simulink model "carac_RPM"  (R2022b)
settings: Solver=VariableStepAuto  StartTime=0.0  StopTime=inf  RelTol=1e-3
libraries: robotlib x3
settings Model: Creator=guillermo  LastModifiedBy=alex

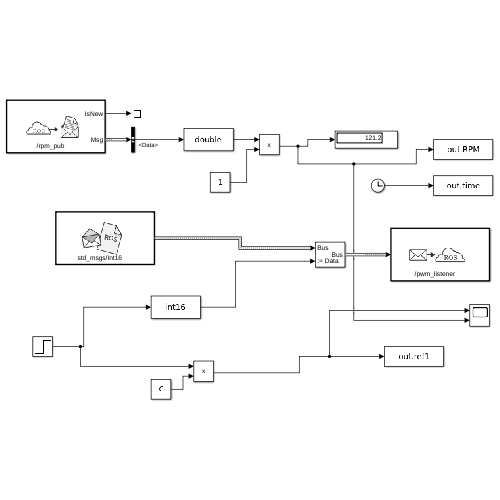
[thumbnail: Simulink's stored preview of the top-level diagram]
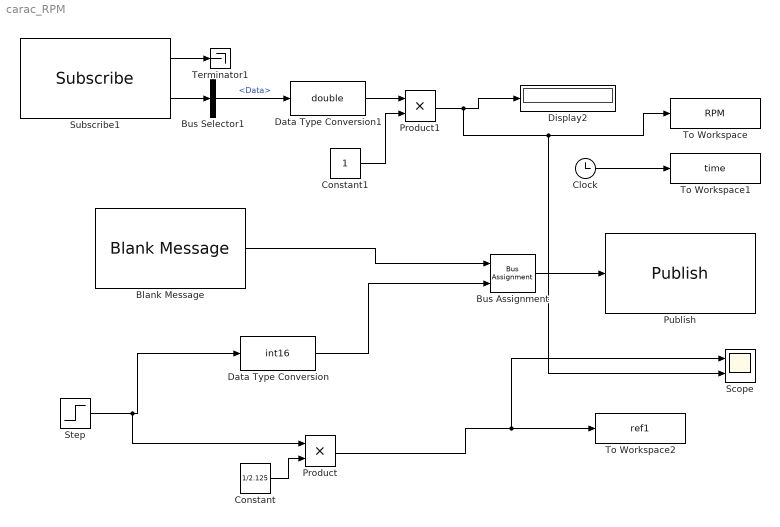
== system carac_RPM ==
  Blank Message : robotlib/Blank Message  messageClass=Message  entityType=std_msgs/Int16  messageType=std_msgs/Int16  SampleTime=inf  legacyBusStruct=off
      settings: LibrarySourceBlock=roslib/ROS/Blank Message
  Bus Assignment : BusAssignment  AssignedSignals=Data
  Bus Selector1 : BusSelector  OutputSignals=Data
  Clock : Clock
  Constant : Constant  Value=1/2.125
  Constant1 : Constant
  Data Type Conversion : DataTypeConversion  OutDataTypeStr=int16  SaturateOnIntegerOverflow=off  RndMeth=Floor
  Data Type Conversion1 : DataTypeConversion  OutDataTypeStr=double  SaturateOnIntegerOverflow=off  RndMeth=Floor
  Display2 : Display
  Product : Product
  Product1 : Product
  Publish : robotlib/Publish  topicSource=Select from ROS network  topic=/pwm_listener  messageType=std_msgs/Int16  legacyBusStruct=off  messageQueueLength=1
      settings: LibrarySourceBlock=roslib/ROS/Publish
  Scope : Scope  NumInputPorts=2
  Step : Step  After=255  SampleTime=0
  Subscribe1 : robotlib/Subscribe  topicSource=Select from ROS network  topic=/rpm_pub  messageType=std_msgs/Float32  SampleTime=-1  legacyBusStruct=off  messageQueueLength=1
      settings: LibrarySourceBlock=roslib/ROS/Subscribe
  Terminator1 : Terminator
  To Workspace : ToWorkspace  VariableName=RPM  SaveFormat=Timeseries  SampleTime=1e-2
  To Workspace1 : ToWorkspace  VariableName=time  SaveFormat=Timeseries  SampleTime=1e-2
  To Workspace2 : ToWorkspace  VariableName=ref1  SaveFormat=Timeseries  SampleTime=-1
  wires:
  Bus Selector1/1 -> Data Type Conversion1/1  "<Data>"
  Subscribe1/1 -> Terminator1/1
  Subscribe1/2 -> Bus Selector1/1
  Blank Message/1 -> Bus Assignment/1
  Bus Assignment/1 -> Publish/1
  Data Type Conversion/1 -> Bus Assignment/2
  Clock/1 -> To Workspace1/1
  Product1/1 -> Scope/2, To Workspace/1, Display2/1
  Data Type Conversion1/1 -> Product1/1
  Constant1/1 -> Product1/2
  Step/1 -> Product/1, Data Type Conversion/1
  Constant/1 -> Product/2
  Product/1 -> Scope/1, To Workspace2/1
